simulink model "Regelkreis_ZK"  (R2021a)
settings: Solver=ode23s  StartTime=0.0  StopTime=2.5  FixedStep=0.0001  MaxStep=1e-3  RelTol=1e-3  EnableMultiTasking=on
values from neighbouring files (symbols this model uses):
  friction_gain = 5.55028e-07    [params_m.m]    (also in strecke_params_m.m = 6e-07)
  I_max_stat = 0.58    [params_m.m]
  J = Jk    (= 7e-07)    [params_m.m]    (also in strecke_params_m.m = 1e-06)
  k_ADC = 1023/5    (= 204.6)    [params_m.m]
  k_cond_i_k = -1/0.1 * 1/4    (= -2.5)    [params_m.m]
  k_cond_i_T = 2.2e-3    (= 0.0022)    [params_m.m]
  k_cond_n_k = -2/1000 * 0.16    (= -0.00032)    [params_m.m]
  k_cond_n_T = 4.7e-3    (= 0.0047)    [params_m.m]
  k_cond_pos = -400/(2*pi)    (= -63.6619772368)    [params_m.m]
  k_cond_pwm_k = -5/255*2    (= -0.0392156862745)    [params_m.m]
  k_cond_pwm_T1 = 340e-6    (= 0.00034)    [params_m.m]
  k_cond_pwm_T2 = 400e-6    (= 0.0004)    [params_m.m]
  k_HPS_u = 12/5    (= 2.4)    [params_m.m]
  km = 14.8e-3    (= 0.0148)    [params_m.m]    (also in strecke_params_m.m)
  L = 2e-3    (= 0.002)    [params_m.m]    (also in strecke_params_m.m)
  n_max = 7800    [params_m.m]
  omega_AW = 0    [params_m.m]    (also in strecke_params_m.m)
  phi_AW = 0 * pi / 180    (= 0)    [params_m.m]    (also in strecke_params_m.m)
  R = 11.9    [params_m.m]    (also in strecke_params_m.m)
  R_shunt = 1.0    (= 1)    [params_m.m]    (also in strecke_params_m.m)
  T_thermisch = 3    [params_m.m]
  u_pwm_a = 220    [params_m.m]
  u_pwm_e = 180    [params_m.m]
libraries: simulink x4, Regler x2
settings Model: Creator=Walter Lindermeir  LastModifiedBy=maowit00
settings SolverCC: AlgebraicLoopSolver=TrustRegion
settings DataIOCC: LimitDataPoints=on  SaveFormat=Array  ReturnWorkspaceOutputs=off
settings OptimizationCC: ExpressionDepthLimit=2147483647  EfficientFloat2IntCast=on  LifeSpan=inf
settings DebuggingCC: SaveWithParameterizedLinksMsg=none  SolverPrmCheckMsg=warning  ParameterTunabilityLossMsg=error  AllowSymbolicDim=off  StateNameClashWarn=warning  StrictBusMsg=ErrorOnBusTreatedAsVector  SFUnexpectedBacktrackingDiag=warning  SFNoUnconditionalDefaultTransitionDiag=warning  SFExecutionAtInitializationDiag=none  SFMachineParentedDataDiag=warning  ArithmeticOperatorsInVariantConditions=warning
settings HardwareCC: ProdBitPerPointer=32  ProdBitPerSizeT=32  ProdBitPerPtrDiffT=32  ProdLargestAtomicFloat=None  ProdIntDivRoundTo=Undefined  ProdEndianess=Unspecified  ProdWordSize=32  ProdHWDeviceType=32-bit Generic
settings ModelReferenceCC: PropagateSignalLabelsOutOfModel=off
settings SFSimCC: SimUseLocalCustomCode=off  CustomCodeUndefinedFunction=UseInterfaceOnly
settings RTWCC: RTWUseLocalCustomCode=off
settings CodeAppCC: StateflowObjectComments=on
settings GRTTargetCC: TargetFcnLib=ansi_tfl_tmw.mat  TargetLangStandard=C89/C90 (ANSI)  CombineOutputUpdateFcns=off  GRTInterface=on
settings ConfigComp: CovMetricSettings=dw  CovSaveCumulativeToWorkspaceVar=on  CovSaveSingleToWorkspaceVar=on  CovExternalEMLEnable=off

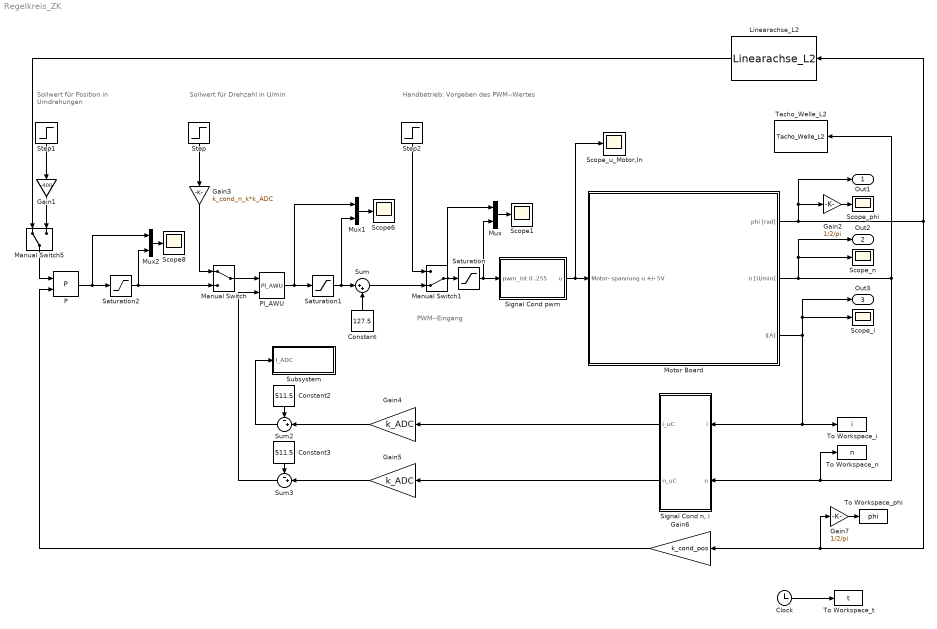
== system Regelkreis_ZK ==
  note: PWM--Eingang
  note: Sollwert für Position
      | in Umdrehungen
  note: Handbetrieb:
      | Vorgeben des PWM--Wertes
  note: Sollwert für Drehzahl
      | in U/min
  Clock : Clock
  Constant : Constant  Value=127.5
  Constant2 : Constant  Value=511.5
  Constant3 : Constant  Value=511.5
  Gain1 : Gain  Gain=-400
  Gain2 : Gain  Gain=1/2/pi
  Gain3 : Gain  Gain=k_cond_n_k*k_ADC
  Gain4 : Gain  Gain=k_ADC
  Gain5 : Gain  Gain=k_ADC
  Gain6 : Gain  Gain=k_cond_pos
  Gain7 : Gain  Gain=1/2/pi
  Linearachse_L2 : M-S-Function  FunctionName=Linearachse_L2  Parameters=enable,ts,phiMax,spindelsteigung  mask(Linearachse){enable=on, ts=0.005, phiMax=15*2*pi, spindelsteigung=5}
      mask prompts: ts "Abtastzeit für Animation"; phiMax "Winkelberich phiMax"; spindelsteigung "Spindelsteigung: Weg pro Umdrehung [mm/U]"
      mask help: Animation einer Linearachse zur Überführung eines Winkels der Welle in eine Position auf einer Linearachse
      mask Display: image('Linearachse.png')
  Manual Switch : ManualSwitch
  Manual Switch1 : ManualSwitch  CurrentSetting=0
  Manual Switch5 : ManualSwitch
  Motor Board : Subsystem
      mask Display: image('HPS.jpg')
  Mux : Mux  Inputs=2
  Mux1 : Mux  Inputs=2
  Mux2 : Mux  Inputs=2
  P : Regler/P  kp=k_Rpos
  PI_AWU : Regler/PI_AWU  kp=k_Rn  Tn=Tn_n  bo=127.5  bu=-127.5
  Saturation : Saturate  UpperLimit=255  LowerLimit=0
  Saturation1 : Saturate  UpperLimit=127.5  LowerLimit=-127.5  ZeroCross=off
  Saturation2 : Saturate  UpperLimit=-n_max*k_cond_n_k*k_ADC  LowerLimit=n_max*k_cond_n_k*k_ADC
  Scope1 : Scope
  Scope6 : Scope
  Scope8 : Scope
  Scope_i : Scope
  Scope_n : Scope
  Scope_phi : Scope
  Scope_u_Motor,In : Scope
  "Signal Cond n, i" : Subsystem
  Signal Cond pwm : Subsystem
  Step : Step  Before=1000  After=3000  SampleTime=0
  Step1 : Step  After=10  SampleTime=0
  Step2 : Step  Before=u_pwm_a  After=u_pwm_e  SampleTime=0
  Subsystem : Subsystem
      mask Display: disp('I2dt check')
  Sum : Sum  Inputs=|++
  Sum2 : Sum  Inputs=-+|
  Sum3 : Sum  Inputs=-+|
  Tacho_Welle_L2 : M-S-Function  FunctionName=Tacho_Welle_L2  Parameters=enable, ts, minimum, maximum, teilung,k  mask{enable=on, ts=0.005, minimum=-8000, maximum=+8000, teilung=1000, k=1}
      mask prompts: ts "Abtastzeit"; minimum "Minimalwert"; maximum "Maximalwert"; teilung "Skalenteilung"; k "Skalierungsfaktor"
      mask Display: image('Tacho_Welle.png');
  To Workspace_i : ToWorkspace  VariableName=i  SampleTime=-1
  To Workspace_n : ToWorkspace  VariableName=n  SampleTime=-1
  To Workspace_phi : ToWorkspace  VariableName=phi  SampleTime=-1
  To Workspace_t : ToWorkspace  VariableName=t  SampleTime=-1
  Out1 : Outport  VectorParamsAs1DForOutWhenUnconnected=off
  Out2 : Outport  Port=2  VectorParamsAs1DForOutWhenUnconnected=off
  Out3 : Outport  Port=3  VectorParamsAs1DForOutWhenUnconnected=off
  wires:
  Saturation/1 -> Mux/2, Signal Cond pwm/1(pwm_int 0..255)
  Manual Switch/1 -> PI_AWU/1
  P/1 -> Saturation2/1, Mux2/1
  Mux/1 -> Scope1/1
  Constant/1 -> Sum/2
  Sum3/1 -> PI_AWU/2
  Constant2/1 -> Sum2/1
  Constant3/1 -> Sum3/1
  Motor Board/1(phi [rad]) -> Gain2/1, Out1/1, Linearachse_L2/1, Gain6/1, Gain7/1
  Motor Board/2(n [U/min]) -> Out2/1, Scope_n/1, Tacho_Welle_L2/1, "Signal Cond n, i"/2(n), To Workspace_n/1
  Saturation1/1 -> Sum/1, Mux1/2
  Mux1/1 -> Scope6/1
  Saturation2/1 -> Manual Switch/2, Mux2/2
  Mux2/1 -> Scope8/1
  Step1/1 -> Gain1/1
  Step/1 -> Gain3/1
  Signal Cond pwm/1(u) -> Scope_u_Motor,In/1, Motor Board/1(Motor- spannung u +/- 5V)
  Sum/1 -> Manual Switch1/2
  Step2/1 -> Manual Switch1/1
  Gain3/1 -> Manual Switch/1
  PI_AWU/1 -> Saturation1/1, Mux1/1
  Gain1/1 -> Manual Switch5/2
  Gain4/1 -> Sum2/2
  Gain5/1 -> Sum3/2
  Gain6/1 -> P/2
  "Signal Cond n, i"/1(i_uC) -> Gain4/1
  "Signal Cond n, i"/2(n_uC) -> Gain5/1
  Manual Switch1/1 -> Saturation/1, Mux/1
  Clock/1 -> To Workspace_t/1
  Gain7/1 -> To Workspace_phi/1
  Motor Board/3(i[A]) -> "Signal Cond n, i"/1(i), To Workspace_i/1, Out3/1, Scope_i/1
  Manual Switch5/1 -> P/1
  Linearachse_L2/1 -> Manual Switch5/1
  Sum2/1 -> Subsystem/1(I_ADC)
  Gain2/1 -> Scope_phi/1

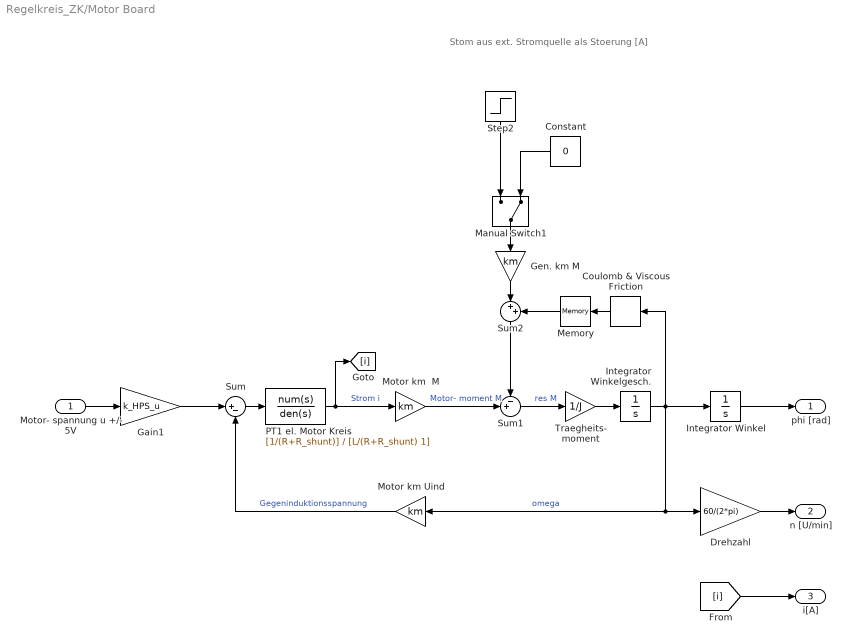
== system Regelkreis_ZK/Motor Board ==
  note: Stom aus ext. Stromquelle
      | als Stoerung [A]
  Motor- spannung u +/- 5V : Inport
  Constant : Constant  Value=0
  Coulomb & Viscous Friction : simulink/Discontinuities/Coulomb & Viscous Friction  offset=friction_offset  gain=friction_gain
  Drehzahl : Gain  Gain=60/(2*pi)
  Gain1 : Gain  Gain=k_HPS_u
  Gen. km M : Gain  Gain=km
  Integrator Winkel : Integrator  InitialCondition=phi_AW
  Integrator Winkelgesch. : Integrator  InitialCondition=omega_AW
  Manual Switch1 : ManualSwitch  CurrentSetting=0
  Memory : Memory  LinearizeMemory=on
  Motor km  M : Gain  Gain=km
  Motor km Uind : Gain  Gain=km
  PT1 el. Motor Kreis : TransferFcn  Numerator=[1/(R+R_shunt)]  Denominator=[L/(R+R_shunt) 1]
  Step2 : Step  Time=2  After=-0.2  SampleTime=0
  Sum : Sum  Inputs=|+-
  Sum1 : Sum  Inputs=-+|
  Sum2 : Sum  Inputs=|++
  Traegheits- moment : Gain  Gain=1/J
  phi [rad] : Outport  VectorParamsAs1DForOutWhenUnconnected=off
  n [U/min] : Outport  Port=2  VectorParamsAs1DForOutWhenUnconnected=off
  i[A] : Outport  Port=3  VectorParamsAs1DForOutWhenUnconnected=off
  wires:
  PT1 el. Motor Kreis/1 -> [i], Motor km  M/1  "Strom i"
  Motor km  M/1 -> Sum1/2  "Motor- moment M"
  Integrator Winkelgesch./1 -> Motor km Uind/1, Drehzahl/1, Coulomb & Viscous Friction/1, Integrator Winkel/1  "omega"
  Integrator Winkel/1 -> phi [rad]/1
  Drehzahl/1 -> n [U/min]/1
  [i] -> i[A]/1
  Gen. km M/1 -> Sum2/1
  Gain1/1 -> Sum/1
  Motor km Uind/1 -> Sum/2  "Gegeninduktionsspannung"
  Sum2/1 -> Sum1/1
  Coulomb & Viscous Friction/1 -> Memory/1
  Memory/1 -> Sum2/2
  Manual Switch1/1 -> Gen. km M/1
  Step2/1 -> Manual Switch1/1
  Constant/1 -> Manual Switch1/2
  Motor- spannung u +/- 5V/1 -> Gain1/1
  Sum/1 -> PT1 el. Motor Kreis/1
  Sum1/1 -> Traegheits- moment/1  "res M"
  Traegheits- moment/1 -> Integrator Winkelgesch./1

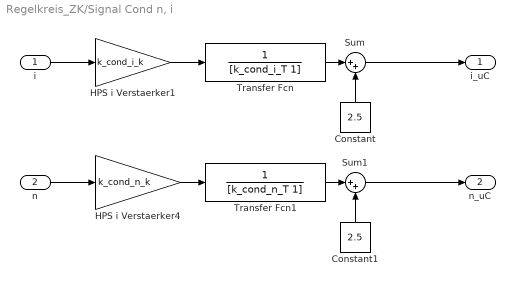
== system Regelkreis_ZK/Signal Cond n, i ==
  i : Inport
  n : Inport  Port=2
  Constant : Constant  Value=2.5
  Constant1 : Constant  Value=2.5
  HPS i Verstaerker1 : Gain  Gain=k_cond_i_k
  HPS i Verstaerker4 : Gain  Gain=k_cond_n_k
  Sum : Sum  Inputs=|++
  Sum1 : Sum  Inputs=|++
  Transfer Fcn : TransferFcn  Denominator=[k_cond_i_T 1]
  Transfer Fcn1 : TransferFcn  Denominator=[k_cond_n_T 1]
  i_uC : Outport  VectorParamsAs1DForOutWhenUnconnected=off
  n_uC : Outport  Port=2  VectorParamsAs1DForOutWhenUnconnected=off
  wires:
  HPS i Verstaerker1/1 -> Transfer Fcn/1
  Transfer Fcn/1 -> Sum/1
  Constant/1 -> Sum/2
  Sum/1 -> i_uC/1
  HPS i Verstaerker4/1 -> Transfer Fcn1/1
  Transfer Fcn1/1 -> Sum1/1
  Constant1/1 -> Sum1/2
  Sum1/1 -> n_uC/1
  i/1 -> HPS i Verstaerker1/1
  n/1 -> HPS i Verstaerker4/1

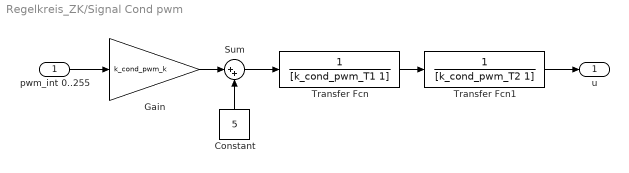
== system Regelkreis_ZK/Signal Cond pwm ==
  pwm_int 0..255 : Inport
  Constant : Constant  Value=5
  Gain : Gain  Gain=k_cond_pwm_k
  Sum : Sum  Inputs=|++
  Transfer Fcn : TransferFcn  Denominator=[k_cond_pwm_T1 1]
  Transfer Fcn1 : TransferFcn  Denominator=[k_cond_pwm_T2 1]
  u : Outport  VectorParamsAs1DForOutWhenUnconnected=off
  wires:
  pwm_int 0..255/1 -> Gain/1
  Gain/1 -> Sum/1
  Constant/1 -> Sum/2
  Transfer Fcn/1 -> Transfer Fcn1/1
  Sum/1 -> Transfer Fcn/1
  Transfer Fcn1/1 -> u/1

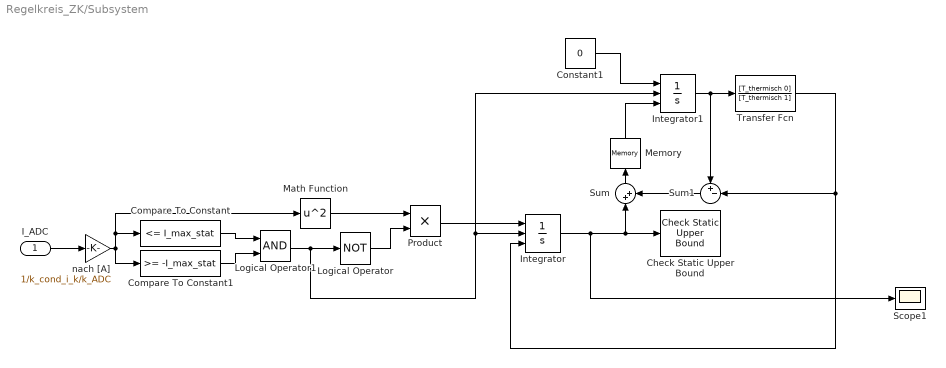
== system Regelkreis_ZK/Subsystem ==
  I_ADC : Inport
  Check Static Upper Bound : simulink/Model Verification/Check Static  Upper Bound  Description=u <= I2dt_max  max=I2dt_max  max_included=on  enabled=on  stopWhenAssertionFail=on  export=off  icon=graphic
      settings: SourceProductBaseCode=SL
  Compare To Constant : simulink/Logic and Bit Operations/Compare To Constant  relop=<=  const=I_max_stat  OutDataTypeStr=boolean  ZeroCross=off
  Compare To Constant1 : simulink/Logic and Bit Operations/Compare To Constant  relop=>=  const=-I_max_stat  OutDataTypeStr=boolean  ZeroCross=off
  Constant1 : Constant  Value=0
  Integrator : Integrator  ExternalReset=level  InitialConditionSource=external  AbsoluteTolerance=1  ZeroCross=off
  Integrator1 : Integrator  ExternalReset=rising  InitialConditionSource=external
  Logical Operator : Logic  Operator=NOT  AllPortsSameDT=off  OutDataTypeStr=uint(8)
  Logical Operator1 : Logic  AllPortsSameDT=off  OutDataTypeStr=boolean
  Math Function : Math  Operator=square  SignedPower=on  SaturateOnIntegerOverflow=on
  Memory : Memory
  Product : Product  RndMeth=Zero
  Scope1 : Scope
  Sum : Sum  Inputs=|++
  Sum1 : Sum  Inputs=+-|
  Transfer Fcn : TransferFcn  Numerator=[T_thermisch 0]  Denominator=[T_thermisch 1]
  nach [A] : Gain  Gain=1/k_cond_i_k/k_ADC
  wires:
  nach [A]/1 -> Compare To Constant/1, Math Function/1, Compare To Constant1/1
  Logical Operator1/1 -> Logical Operator/1, Integrator/2, Integrator1/2
  Logical Operator/1 -> Product/2
  Integrator/1 -> Sum/1, Check Static Upper Bound/1, Scope1/1
  I_ADC/1 -> nach [A]/1
  Compare To Constant/1 -> Logical Operator1/1
  Compare To Constant1/1 -> Logical Operator1/2
  Math Function/1 -> Product/1
  Transfer Fcn/1 -> Sum1/2, Integrator/3
  Product/1 -> Integrator/1
  Constant1/1 -> Integrator1/1
  Integrator1/1 -> Transfer Fcn/1, Sum1/1
  Sum/1 -> Memory/1
  Memory/1 -> Integrator1/3
  Sum1/1 -> Sum/2
